simulink model "DGM_test_sim"  (R2020a)
settings: Solver=VariableStepAuto  StartTime=0.0  StopTime=smax  MaxStep=0.01  RelTol=1e-3
values from neighbouring files (symbols this model uses):
  a1 = 2    [OvereniDGMIGM.m]    (also in setup.m)
  a2 = 1.5    [OvereniDGMIGM.m]    (also in setup.m)
  a3 = 0.5    [OvereniDGMIGM.m]    (also in setup.m)
  T_1_0 = [cos(theta10), -sin(theta10), 0, a1*cos(theta10) ... (first row only)    [OvereniDGMIGM.m]    (also in setup.m)
  T_2_1 = [cos(theta20), -sin(theta20), 0, a2*cos(theta20) ... (first row only)    [OvereniDGMIGM.m]    (also in setup.m)
  T_3_2 = [cos(theta30), -sin(theta30), 0, a3*cos(theta30) ... (first row only)    [OvereniDGMIGM.m]    (also in setup.m)
undefined symbols (not defined in the file or in its folder): fi_s, fi_sample, r, R, smax, X, Y, Z
libraries: sm_lib x114, nesl_utility x58, simulink x4
(part 4 of 4)

== matlab function DGM_test_sim/MATLAB Function7 ==
  data: theta1 input; theta2 input; theta3 input; theta1_dot input; theta2_dot input; theta3_dot input; theta1_dot_dot input; theta2_dot_dot input; theta3_dot_dot input; a1 parameter; a2 parameter; a3 parameter; x output; y output; phi output; dx output; dy output; dphi output; ddx output; ddy output; ddphi output
function [ x, y, phi, dx, dy, dphi, ddx, ddy, ddphi] = POKU(theta1,theta2, theta3, theta1_dot,theta2_dot,theta3_dot,theta1_dot_dot,theta2_dot_dot,theta3_dot_dot,a1,a2,a3)
    % poloha
%     
    position = NaN(3,1);
    position(1) = a3*cos(theta1+theta2+theta3) + a2*cos(theta1+theta2) + a1*cos(theta1);
    position(2) = a3*sin(theta1+theta2+theta3) + a2*sin(theta1+theta2) + a1*sin(theta1);
    position(3) = atan2(sin(theta1+theta2+theta3),cos(theta1+theta2+theta3));
   
    % rychlost
    JQ = [-a3 * sin(theta1 + theta2 + theta3) - a2 * sin(theta1 + theta2) - a1 * sin(theta1), -a3 * sin(theta1 + theta2 + theta3) - a2 * sin(theta1 + theta2), -a3 * sin(theta1 + theta2 + theta3);
           a3 * cos(theta1 + theta2 + theta3) + a2 * cos(theta1 + theta2) + a1 * cos(theta1), a3 * cos(theta1 + theta2 + theta3) + a2 * cos(theta1 + theta2), a3 * cos(theta1 + theta2 + theta3);
          1,1,1];
    theta_dot = [theta1_dot, theta2_dot, theta3_dot]';
    theta_dot_123 = theta1_dot + theta2_dot + theta3_dot;
    theta_dot_12 = theta1_dot + theta2_dot;
    speed = JQ * theta_dot;
    
    % zrychlenis
    dJQ = [-a3 * cos(theta1 + theta1 + theta1) * theta_dot_123 - a2 * cos(theta1 + theta2) * theta_dot_12 - a1 * cos(theta1)*theta1_dot, - a3*cos(theta1 + theta2 + theta3) * theta_dot_123 - a2*cos(theta1 + theta2) * theta_dot_12, -a3 * cos(theta1 + theta2 + theta3) * theta_dot_123;
       -a3 * sin(theta1 + theta2 + theta3) * theta_dot_123 - a2 * sin(theta1 + theta2) * theta_dot_12 - a1 * sin(theta1)*theta1_dot, - a3*sin(theta1 + theta2 + theta3) * theta_dot_123 - a2*sin(theta1 + theta2) * theta_dot_12, -a3 * sin(theta1 + theta2 + theta3) * theta_dot_123;
       0,0,0];
    theta_dot_dot = [theta1_dot_dot, theta2_dot_dot, theta3_dot_dot]';

    acceleration = dJQ * theta_dot + JQ * theta_dot_dot;
    
    x = position(1);
    y = position(2);
    phi = position(3);
    dx = speed(1);
    dy = speed(2);
    dphi = speed(3);
    ddx = acceleration(1);
    ddy = acceleration(2);
    ddphi = acceleration(3);
    
end

== matlab function DGM_test_sim/MATLAB Function8 ==
  data: x input; y input; phi input; dx input; dy input; dphi input; ddx input; ddy input; ddphi input; a1 parameter; a2 parameter; a3 parameter; theta1 output size=1; theta2 output size=1; theta3 output size=1; theta1_dot output size=1; theta2_dot output size=1; theta3_dot output size=1; theta1_dot_dot output size=1; theta2_dot_dot output size=1; theta3_dot_dot output size=1
function [theta1, theta2, theta3,theta1_dot,theta2_dot,theta3_dot,theta1_dot_dot,theta2_dot_dot,theta3_dot_dot] = IOKU( x, y, phi, dx, dy, dphi, ddx, ddy, ddphi, a1, a2, a3)

% theta2
cosQ2 = ((x - a3*cos(phi))^2 + (y - a3*sin(phi))^2 - a1^2 - a2^2)/(2 * a1 * a2);
sinQ2 = -abs(sqrt(abs(1 - cosQ2^2)));
theta2 = atan2(sinQ2, cosQ2);

% theta1
A = [-a2 * sinQ2, a2 * cosQ2 + a1; a2 * cosQ2 + a1, a2 * sinQ2];
B = [x - a3*cos(phi); y - a3*sin(phi)];
X = A\B;
theta1 = atan2(X(1), X(2));

% theta3
theta3 = phi - theta1 - theta2;

% uhlova rychlost
JQ = [-a3 * sin(theta1 + theta2 + theta3) - a2 * sin(theta1 + theta2) - a1 * sin(theta1), -a3 * sin(theta1 + theta2 + theta3) - a2 * sin(theta1 + theta2), -a3 * sin(theta1 + theta2 + theta3);...
       a3 * cos(theta1 + theta2 + theta3) + a2 * cos(theta1 + theta2) + a1 * cos(theta1), a3 * cos(theta1 + theta2 + theta3) + a2 * cos(theta1 + theta2), a3 * cos(theta1 + theta2 + theta3);...
       1, 1, 1];
dX = [dx; dy; dphi];
dQ = JQ^(-1) * dX;
theta1_dot = dQ(1);
theta2_dot = dQ(2);
theta3_dot = dQ(3);

% uhlove zrychleni
dJQ = [-a3*cos(theta1+theta2+theta3)*(theta1_dot+theta2_dot+theta3_dot) - a2*cos(theta1+theta2)*(theta1_dot+theta2_dot) - a1*cos(theta1)*theta1_dot, -a3*cos(theta1+theta2+theta3)*(theta1_dot+theta2_dot+theta3_dot) - a2*cos(theta1+theta2)*(theta1_dot+theta2_dot), -a3*cos(theta1+theta2+theta3)*(theta1_dot+theta2_dot+theta3_dot);...
    -a3*sin(theta1+theta2+theta3)*(theta1_dot+theta2_dot+theta3_dot) - a2*sin(theta1+theta2)*(theta1_dot+theta2_dot) - a1*sin(theta1)*theta1_dot, -a3*sin(theta1+theta2+theta3)*(theta1_dot+theta2_dot+theta3_dot) - a2*sin(theta1+theta2)*(theta1_dot+theta2_dot), -a3*sin(theta1+theta2+theta3)*(theta1_dot+theta2_dot+theta3_dot);...
    0, 0, 0];
ddX = [ddx; ddy; ddphi];
ddQ = JQ^(-1) * (ddX - dJQ * dQ);
theta1_dot_dot = ddQ(1);
theta2_dot_dot = ddQ(2);
theta3_dot_dot = ddQ(3);


end

== matlab function DGM_test_sim/MATLAB Function10 ==
  data: x input; y input; phi input; dx input; dy input; dphi input; ddx input; ddy input; ddphi input; a1 parameter; a2 parameter; a3 parameter; theta1 output size=1; theta2 output size=1; theta3 output size=1; theta1_dot output size=1; theta2_dot output size=1; theta3_dot output size=1; theta1_dot_dot output size=1; theta2_dot_dot output size=1; theta3_dot_dot output size=1
function [theta1, theta2, theta3,theta1_dot,theta2_dot,theta3_dot,theta1_dot_dot,theta2_dot_dot,theta3_dot_dot] = IOKU( x, y, phi, dx, dy, dphi, ddx, ddy, ddphi, a1, a2, a3)

% theta2
cosQ2 = ((x - a3*cos(phi))^2 + (y - a3*sin(phi))^2 - a1^2 - a2^2)/(2 * a1 * a2);
sinQ2 = -abs(sqrt(abs(1 - cosQ2^2)));
theta2 = atan2(sinQ2, cosQ2);

% theta1
A = [-a2 * sinQ2, a2 * cosQ2 + a1; a2 * cosQ2 + a1, a2 * sinQ2];
B = [x - a3*cos(phi); y - a3*sin(phi)];
X = A\B;
theta1 = atan2(X(1), X(2));

% theta3
theta3 = phi - theta1 - theta2;

% uhlova rychlost
JQ = [-a3 * sin(theta1 + theta2 + theta3) - a2 * sin(theta1 + theta2) - a1 * sin(theta1), -a3 * sin(theta1 + theta2 + theta3) - a2 * sin(theta1 + theta2), -a3 * sin(theta1 + theta2 + theta3);...
       a3 * cos(theta1 + theta2 + theta3) + a2 * cos(theta1 + theta2) + a1 * cos(theta1), a3 * cos(theta1 + theta2 + theta3) + a2 * cos(theta1 + theta2), a3 * cos(theta1 + theta2 + theta3);...
       1, 1, 1];
dX = [dx; dy; dphi];
dQ = JQ^(-1) * dX;
theta1_dot = dQ(1);
theta2_dot = dQ(2);
theta3_dot = dQ(3);

% uhlove zrychleni
dJQ = [-a3*cos(theta1+theta2+theta3)*(theta1_dot+theta2_dot+theta3_dot) - a2*cos(theta1+theta2)*(theta1_dot+theta2_dot) - a1*cos(theta1)*theta1_dot, -a3*cos(theta1+theta2+theta3)*(theta1_dot+theta2_dot+theta3_dot) - a2*cos(theta1+theta2)*(theta1_dot+theta2_dot), -a3*cos(theta1+theta2+theta3)*(theta1_dot+theta2_dot+theta3_dot);...
    -a3*sin(theta1+theta2+theta3)*(theta1_dot+theta2_dot+theta3_dot) - a2*sin(theta1+theta2)*(theta1_dot+theta2_dot) - a1*sin(theta1)*theta1_dot, -a3*sin(theta1+theta2+theta3)*(theta1_dot+theta2_dot+theta3_dot) - a2*sin(theta1+theta2)*(theta1_dot+theta2_dot), -a3*sin(theta1+theta2+theta3)*(theta1_dot+theta2_dot+theta3_dot);...
    0, 0, 0];
ddX = [ddx; ddy; ddphi];
ddQ = JQ^(-1) * (ddX - dJQ * dQ);
theta1_dot_dot = ddQ(1);
theta2_dot_dot = ddQ(2);
theta3_dot_dot = ddQ(3);


end

== matlab function DGM_test_sim/MATLAB Function9 ==
  data: theta1 input; theta2 input; theta3 input; theta1_dot input; theta2_dot input; theta3_dot input; theta1_dot_dot input; theta2_dot_dot input; theta3_dot_dot input; a1 parameter; a2 parameter; a3 parameter; x output; y output; phi output; dx output; dy output; dphi output; ddx output; ddy output; ddphi output
function [ x, y, phi, dx, dy, dphi, ddx, ddy, ddphi] = POKU(theta1,theta2, theta3, theta1_dot,theta2_dot,theta3_dot,theta1_dot_dot,theta2_dot_dot,theta3_dot_dot,a1,a2,a3)
    % poloha
%     
    position = NaN(3,1);
    position(1) = a3*cos(theta1+theta2+theta3) + a2*cos(theta1+theta2) + a1*cos(theta1);
    position(2) = a3*sin(theta1+theta2+theta3) + a2*sin(theta1+theta2) + a1*sin(theta1);
    position(3) = atan2(sin(theta1+theta2+theta3),cos(theta1+theta2+theta3));
   
    % rychlost
    JQ = [-a3 * sin(theta1 + theta2 + theta3) - a2 * sin(theta1 + theta2) - a1 * sin(theta1), -a3 * sin(theta1 + theta2 + theta3) - a2 * sin(theta1 + theta2), -a3 * sin(theta1 + theta2 + theta3);
           a3 * cos(theta1 + theta2 + theta3) + a2 * cos(theta1 + theta2) + a1 * cos(theta1), a3 * cos(theta1 + theta2 + theta3) + a2 * cos(theta1 + theta2), a3 * cos(theta1 + theta2 + theta3);
          1,1,1];
    theta_dot = [theta1_dot, theta2_dot, theta3_dot]';
    theta_dot_123 = theta1_dot + theta2_dot + theta3_dot;
    theta_dot_12 = theta1_dot + theta2_dot;
    speed = JQ * theta_dot;
    
    % zrychlenis
    dJQ = [-a3 * cos(theta1 + theta2 + theta3) * theta_dot_123 - a2 * cos(theta1 + theta2) * theta_dot_12 - a1 * cos(theta1)*theta1_dot, - a3*cos(theta1 + theta2 + theta3) * theta_dot_123 - a2*cos(theta1 + theta2) * theta_dot_12, -a3 * cos(theta1 + theta2 + theta3) * theta_dot_123;
       -a3 * sin(theta1 + theta2 + theta3) * theta_dot_123 - a2 * sin(theta1 + theta2) * theta_dot_12 - a1 * sin(theta1)*theta1_dot, - a3*sin(theta1 + theta2 + theta3) * theta_dot_123 - a2*sin(theta1 + theta2) * theta_dot_12, -a3 * sin(theta1 + theta2 + theta3) * theta_dot_123;
       0,0,0];
    theta_dot_dot = [theta1_dot_dot, theta2_dot_dot, theta3_dot_dot]';

    acceleration = dJQ * theta_dot + JQ * theta_dot_dot;
    
    x = position(1);
    y = position(2);
    phi = position(3);
    dx = speed(1);
    dy = speed(2);
    dphi = speed(3);
    ddx = acceleration(1);
    ddy = acceleration(2);
    ddphi = acceleration(3);
    
end

== matlab function DGM_test_sim/MATLAB Function11 ==
  data: x input; y input; phi input; dx input; dy input; dphi input; ddx input; ddy input; ddphi input; a1 parameter; a2 parameter; a3 parameter; theta1 output size=1; theta2 output size=1; theta3 output size=1; theta1_dot output size=1; theta2_dot output size=1; theta3_dot output size=1; theta1_dot_dot output size=1; theta2_dot_dot output size=1; theta3_dot_dot output size=1
function [theta1, theta2, theta3,theta1_dot,theta2_dot,theta3_dot,theta1_dot_dot,theta2_dot_dot,theta3_dot_dot] = IOKU( x, y, phi, dx, dy, dphi, ddx, ddy, ddphi, a1, a2, a3)

% theta2
cosQ2 = ((x - a3*cos(phi))^2 + (y - a3*sin(phi))^2 - a1^2 - a2^2)/(2 * a1 * a2);
sinQ2 = -abs(sqrt(abs(1 - cosQ2^2)));
theta2 = atan2(sinQ2, cosQ2);

% theta1
A = [-a2 * sin(theta2), a2 * cos(theta2) + a1; a2 * cos(theta2) + a1, a2 * sin(theta2)];
B = [x - a3*cos(phi); y - a3*sin(phi)];
X = A\B;
theta1 = atan2(X(1), X(2));

% theta3
theta3 = phi - theta1 - theta2;

% uhlova rychlost
JQ = [-a3 * sin(theta1 + theta2 + theta3) - a2 * sin(theta1 + theta2) - a1 * sin(theta1), -a3 * sin(theta1 + theta2 + theta3) - a2 * sin(theta1 + theta2), -a3 * sin(theta1 + theta2 + theta3);...
       a3 * cos(theta1 + theta2 + theta3) + a2 * cos(theta1 + theta2) + a1 * cos(theta1), a3 * cos(theta1 + theta2 + theta3) + a2 * cos(theta1 + theta2), a3 * cos(theta1 + theta2 + theta3);...
       1, 1, 1];
dX = [dx; dy; dphi];
dQ = JQ^(-1) * dX;
theta1_dot = dQ(1);
theta2_dot = dQ(2);
theta3_dot = dQ(3);

% uhlove zrychleni
dJQ = [-a3*cos(theta1+theta2+theta3)*(theta1_dot+theta2_dot+theta3_dot) - a2*cos(theta1+theta2)*(theta1_dot+theta2_dot) - a1*cos(theta1)*theta1_dot, -a3*cos(theta1+theta2+theta3)*(theta1_dot+theta2_dot+theta3_dot) - a2*cos(theta1+theta2)*(theta1_dot+theta2_dot), -a3*cos(theta1+theta2+theta3)*(theta1_dot+theta2_dot+theta3_dot);...
    -a3*sin(theta1+theta2+theta3)*(theta1_dot+theta2_dot+theta3_dot) - a2*sin(theta1+theta2)*(theta1_dot+theta2_dot) - a1*sin(theta1)*theta1_dot, -a3*sin(theta1+theta2+theta3)*(theta1_dot+theta2_dot+theta3_dot) - a2*sin(theta1+theta2)*(theta1_dot+theta2_dot), -a3*sin(theta1+theta2+theta3)*(theta1_dot+theta2_dot+theta3_dot);...
    0, 0, 0];
ddX = [ddx; ddy; ddphi];
ddQ = JQ^(-1) * (ddX - dJQ * dQ);
theta1_dot_dot = ddQ(1);
theta2_dot_dot = ddQ(2);
theta3_dot_dot = ddQ(3);


end

== matlab function DGM_test_sim/MATLAB Function12 ==
  data: x input; y input; phi input; dx input; dy input; dphi input; ddx input; ddy input; ddphi input; a1 parameter; a2 parameter; a3 parameter; theta1 output size=1; theta2 output size=1; theta3 output size=1; theta1_dot output size=1; theta2_dot output size=1; theta3_dot output size=1; theta1_dot_dot output size=1; theta2_dot_dot output size=1; theta3_dot_dot output size=1
function [theta1, theta2, theta3,theta1_dot,theta2_dot,theta3_dot,theta1_dot_dot,theta2_dot_dot,theta3_dot_dot] = IOKU( x, y, phi, dx, dy, dphi, ddx, ddy, ddphi, a1, a2, a3)

% theta2
cosQ2 = ((x - a3*cos(phi))^2 + (y - a3*sin(phi))^2 - a1^2 - a2^2)/(2 * a1 * a2);
sinQ2 = -abs(sqrt(abs(1 - cosQ2^2)));
theta2 = atan2(sinQ2, cosQ2);

% theta1
A = [-a2 * sin(theta2), a2 * cos(theta2) + a1; a2 * cos(theta2) + a1, a2 * sin(theta2)];
B = [x - a3*cos(phi); y - a3*sin(phi)];
X = A\B;
theta1 = atan2(X(1), X(2));

% theta3
theta3 = phi - theta1 - theta2;

% uhlova rychlost
JQ = [-a3 * sin(theta1 + theta2 + theta3) - a2 * sin(theta1 + theta2) - a1 * sin(theta1), -a3 * sin(theta1 + theta2 + theta3) - a2 * sin(theta1 + theta2), -a3 * sin(theta1 + theta2 + theta3);...
       a3 * cos(theta1 + theta2 + theta3) + a2 * cos(theta1 + theta2) + a1 * cos(theta1), a3 * cos(theta1 + theta2 + theta3) + a2 * cos(theta1 + theta2), a3 * cos(theta1 + theta2 + theta3);...
       1, 1, 1];
dX = [dx; dy; dphi];
dQ = JQ^(-1) * dX;
theta1_dot = dQ(1);
theta2_dot = dQ(2);
theta3_dot = dQ(3);

% uhlove zrychleni
dJQ = [-a3*cos(theta1+theta2+theta3)*(theta1_dot+theta2_dot+theta3_dot) - a2*cos(theta1+theta2)*(theta1_dot+theta2_dot) - a1*cos(theta1)*theta1_dot, -a3*cos(theta1+theta2+theta3)*(theta1_dot+theta2_dot+theta3_dot) - a2*cos(theta1+theta2)*(theta1_dot+theta2_dot), -a3*cos(theta1+theta2+theta3)*(theta1_dot+theta2_dot+theta3_dot);...
    -a3*sin(theta1+theta2+theta3)*(theta1_dot+theta2_dot+theta3_dot) - a2*sin(theta1+theta2)*(theta1_dot+theta2_dot) - a1*sin(theta1)*theta1_dot, -a3*sin(theta1+theta2+theta3)*(theta1_dot+theta2_dot+theta3_dot) - a2*sin(theta1+theta2)*(theta1_dot+theta2_dot), -a3*sin(theta1+theta2+theta3)*(theta1_dot+theta2_dot+theta3_dot);...
    0, 0, 0];
ddX = [ddx; ddy; ddphi];
ddQ = JQ^(-1) * (ddX - dJQ * dQ);
theta1_dot_dot = ddQ(1);
theta2_dot_dot = ddQ(2);
theta3_dot_dot = ddQ(3);


end

== matlab function DGM_test_sim/MATLAB Function ==
  data: s input; Xstar output size=2; v input; a input; dXstar output size=2; ddXstar output size=2
function [Xstar, dXstar, ddXstar] = MCSstar(s, v, a)

    A = [2 0.5]';
    B = [-1 1]'
%     B = [1 1]';
    C = [2 2.5]'
%     sC = -A;

    r = 0.3;
    vmax = 1;
    
    if v > vmax
        v = vmax;
    else
        v = v;
    end
    nba = (A - B)/norm(A-B);
    nbc = (C-B)/norm(C-B);
    nbs = (nba+nbc)/norm(nba+nbc);
    K1 = (nba*nba'*nbs-nbs);
    l = r/(sqrt(K1'*K1));
    S = B+nbs*l;
    k = nba'*(A-S);
    Pa = A-nba*k;
    Pc = B + norm(Pa-B)*nbc;
    
%     
%     x_pab = A-k1.*nba
    Pb = B;

    helper = (Pa-S);
    fi_pa = atan2(helper(2),helper(1));
    dir = -1;
    deltafi = acos(((Pc-S)'*(Pa-S))/r^2);
    
    s1 = norm(Pa-A);
    s2 = norm(Pc-C);
    sk = r*deltafi;
    s1+s2+sk
    if s < s1
        k1 = s;
        dk1 = v;
        ddk1 = a;
        Xstar = A-k1*nba;
        dXstar = -dk1*nba;
        ddXstar = -ddk1*nba;
    elseif s1 <= s &&  s < s1+sk
        Phi = (s-s1)/r;
        dPhi = v/r;
        ddPhi = a/r;
        
        Xstar = r* [cos(fi_pa + dir*Phi); sin(fi_pa + dir*Phi)] + S;
        dXstar = r* [-sin(fi_pa + dir*Phi); cos(fi_pa + dir*Phi)]*dir*dPhi;
        ddXstar = r* [-cos(fi_pa + dir*Phi); -sin(fi_pa + dir*Phi)]*dPhi^2 + r* [-sin(fi_pa + dir*Phi); cos(fi_pa + dir*Phi)]*dir*ddPhi;
    elseif s1+sk < s && s < s1+sk+s2
        k2 = s-s1-sk;
        dk2 = v;
        ddk2 = a;
        
        Xstar = Pc + k2*nbc;
        dXstar = dk2*nbc;
        ddXstar = ddk2*nbc;
    else
%         display('ERROR V TRAJEKTORII')
        Xstar = C;
        dXstar = zeros(2,1);
        ddXstar = zeros(2,1);
    end
   
%     
%     k1 = linspace(0,norm(A-Pa),100)
% 
% 
%     
%     fi = linspace(0,deltafi,100)
%     x_rot = [r*cos(fi_pa+dir*fi);
%              r*sin(fi_pa+dir*fi)]+S
% 
%     k2 = linspace(0,norm(Pc-C),100)
%     x_pbc = Pc + k2.*nbc
% 
% 
% 
%     smax = s1+s2+sk
%     Tmax = smax/vmax
% 
%     T = 100
%     t = linspace(0,Tmax,T)
%     t1 = linspace(0,s1/vmax,T)
%     tk = linspace(s1/vmax,sk/vmax,T)
%     t2 = linspace(sk/vmax,s2/vmax,T)
%     % s = linspace(0,smax,smax/Tmax*10)
%     s = vmax*t
% 
% 
%     k1 = 0+vmax*t
% 
%     k1 = linspace(0,s1,s1/Tmax*T)
%     fi = linspace(0,(sk)/r,(sk)/Tmax*T)
%     k2 = linspace(0,s2,s2/Tmax*T)
% 
%     
%     Xk = [r*cos(fi_pa+dir*fi);r*sin(fi_pa+dir*fi)]+S
%     X2 = Pc+k2.*nbc


end

== matlab function DGM_test_sim/MATLAB Function14 ==
  data: x input; y input; phi input; dx input; dy input; dphi input; ddx input; ddy input; ddphi input; a1 parameter; a2 parameter; a3 parameter; theta1 output size=1; theta2 output size=1; theta3 output size=1; theta1_dot output size=1; theta2_dot output size=1; theta3_dot output size=1; theta1_dot_dot output size=1; theta2_dot_dot output size=1; theta3_dot_dot output size=1
function [theta1, theta2, theta3,theta1_dot,theta2_dot,theta3_dot,theta1_dot_dot,theta2_dot_dot,theta3_dot_dot] = IOKU( x, y, phi, dx, dy, dphi, ddx, ddy, ddphi, a1, a2, a3)

% theta2
cosQ2 = ((x - a3*cos(phi))^2 + (y - a3*sin(phi))^2 - a1^2 - a2^2)/(2 * a1 * a2);
sinQ2 = -abs(sqrt(abs(1 - cosQ2^2)));
theta2 = atan2(sinQ2, cosQ2);

% theta1
A = [-a2 * sin(theta2), a2 * cos(theta2) + a1; a2 * cos(theta2) + a1, a2 * sin(theta2)];
B = [x - a3*cos(phi); y - a3*sin(phi)];
X = A\B;
theta1 = atan2(X(1), X(2));

% theta3
theta3 = phi - theta1 - theta2;

% uhlova rychlost
JQ = [-a3 * sin(theta1 + theta2 + theta3) - a2 * sin(theta1 + theta2) - a1 * sin(theta1), -a3 * sin(theta1 + theta2 + theta3) - a2 * sin(theta1 + theta2), -a3 * sin(theta1 + theta2 + theta3);...
       a3 * cos(theta1 + theta2 + theta3) + a2 * cos(theta1 + theta2) + a1 * cos(theta1), a3 * cos(theta1 + theta2 + theta3) + a2 * cos(theta1 + theta2), a3 * cos(theta1 + theta2 + theta3);...
       1, 1, 1];
dX = [dx; dy; dphi];
dQ = JQ^(-1) * dX;
theta1_dot = dQ(1);
theta2_dot = dQ(2);
theta3_dot = dQ(3);

% uhlove zrychleni
dJQ = [-a3*cos(theta1+theta2+theta3)*(theta1_dot+theta2_dot+theta3_dot) - a2*cos(theta1+theta2)*(theta1_dot+theta2_dot) - a1*cos(theta1)*theta1_dot, -a3*cos(theta1+theta2+theta3)*(theta1_dot+theta2_dot+theta3_dot) - a2*cos(theta1+theta2)*(theta1_dot+theta2_dot), -a3*cos(theta1+theta2+theta3)*(theta1_dot+theta2_dot+theta3_dot);...
    -a3*sin(theta1+theta2+theta3)*(theta1_dot+theta2_dot+theta3_dot) - a2*sin(theta1+theta2)*(theta1_dot+theta2_dot) - a1*sin(theta1)*theta1_dot, -a3*sin(theta1+theta2+theta3)*(theta1_dot+theta2_dot+theta3_dot) - a2*sin(theta1+theta2)*(theta1_dot+theta2_dot), -a3*sin(theta1+theta2+theta3)*(theta1_dot+theta2_dot+theta3_dot);...
    0, 0, 0];
ddX = [ddx; ddy; ddphi];
ddQ = JQ^(-1) * (ddX - dJQ * dQ);
theta1_dot_dot = ddQ(1);
theta2_dot_dot = ddQ(2);
theta3_dot_dot = ddQ(3);


end

== matlab function DGM_test_sim/MATLAB Function15 ==
  data: s input; Xstar output size=2; v input; a input; dXstar output size=2; ddXstar output size=2
function [Xstar, dXstar, ddXstar] = MCSstar(s, v, a)

    A = [2 0.5]';
    B = [0 1]';
%     B = [1 1]';
    C = [2 2.5]';
%     sC = -A;

    r = 0.3;
    vmax = 1;
    
    if v > vmax
        v = vmax;
    else
        v = v;
    end
    nba = (A - B)/norm(A-B);
    nbc = (C-B)/norm(C-B);
    nbs = (nba+nbc)/norm(nba+nbc);
    K1 = (nba*nba'*nbs-nbs);
    l = r/(sqrt(K1'*K1));
    S = B+nbs*l;
    k = nba'*(A-S);
    Pa = A-nba*k;
    Pc = B + norm(Pa-B)*nbc;
    
%     
%     x_pab = A-k1.*nba
    Pb = B;

    helper = (Pa-S);
    fi_pa = atan2(helper(2),helper(1));
    dir = -1;
    deltafi = acos(((Pc-S)'*(Pa-S))/r^2);
    
    s1 = norm(Pa-A);
    s2 = norm(Pc-C);
    sk = r*deltafi;
    s1+s2+sk;
    if s < s1
        k1 = s;
        dk1 = v;
        ddk1 = a;
        Xstar = A-k1*nba;
        dXstar = -dk1*nba;
        ddXstar = -ddk1*nba;
    elseif s1 <= s &&  s < s1+sk
        Phi = (s-s1)/r;
        dPhi = v/r;
        ddPhi = a/r;
        
        Xstar = r* [cos(fi_pa + dir*Phi); sin(fi_pa + dir*Phi)] + S;
        dXstar = r* [-sin(fi_pa + dir*Phi); cos(fi_pa + dir*Phi)]*dir*dPhi;
        ddXstar = r* [-cos(fi_pa + dir*Phi); -sin(fi_pa + dir*Phi)]*dPhi^2 + r* [-sin(fi_pa + dir*Phi); cos(fi_pa + dir*Phi)]*dir*ddPhi;
    elseif s1+sk < s && s < s1+sk+s2
        k2 = s-s1-sk;
        dk2 = v;
        ddk2 = a;
        
        Xstar = Pc + k2*nbc;
        dXstar = dk2*nbc;
        ddXstar = ddk2*nbc;
    else
%         display('ERROR V TRAJEKTORII')
        Xstar = C;
        dXstar = zeros(2,1);
        ddXstar = zeros(2,1);
    end
   
%     
%     k1 = linspace(0,norm(A-Pa),100)
% 
% 
%     
%     fi = linspace(0,deltafi,100)
%     x_rot = [r*cos(fi_pa+dir*fi);
%              r*sin(fi_pa+dir*fi)]+S
% 
%     k2 = linspace(0,norm(Pc-C),100)
%     x_pbc = Pc + k2.*nbc
% 
% 
% 
%     smax = s1+s2+sk
%     Tmax = smax/vmax
% 
%     T = 100
%     t = linspace(0,Tmax,T)
%     t1 = linspace(0,s1/vmax,T)
%     tk = linspace(s1/vmax,sk/vmax,T)
%     t2 = linspace(sk/vmax,s2/vmax,T)
%     % s = linspace(0,smax,smax/Tmax*10)
%     s = vmax*t
% 
% 
%     k1 = 0+vmax*t
% 
%     k1 = linspace(0,s1,s1/Tmax*T)
%     fi = linspace(0,(sk)/r,(sk)/Tmax*T)
%     k2 = linspace(0,s2,s2/Tmax*T)
% 
%     
%     Xk = [r*cos(fi_pa+dir*fi);r*sin(fi_pa+dir*fi)]+S
%     X2 = Pc+k2.*nbc


end

== matlab function DGM_test_sim/MATLAB Function1 ==
  data: theta1 output size=1; x input; theta2 output size=1; y input; phi input; a1 input; a2 input; a3 input; theta3 output size=1
function [theta1, theta2, theta3] = IGM( x, y, phi, a1, a2, a3)
    cosQ2 = ((x - a3 *cos(phi))^2 + (y - a3 * sin(phi))^2 - a2^2 - a1^2)/(2*a1*a2);
    sinQ2 =  -abs(sqrt(abs(1 - cosQ2^2))); % 2 reseni, vybereme -
    
    theta2 = atan2(sinQ2, cosQ2); % Q2
%     A = [-a2 * sin(theta2), a2*cos(theta2) + a1;
%          a2 * cos(theta2)  + a1, a2*sin(theta2)];
     A = [-a2 * sinQ2, a2*cosQ2 + a1;
         a2 * cosQ2  + a1, a2*sinQ2];
    b = [x - a3 * cos(phi); y - a3 * sin(phi)];
    
    X = inv(A)*b;
%     sin(theta1) = X(1);
%     cos(theta1) = X(2);
    
    theta1 = atan2(X(1),X(2)); % Q1
    
    theta3 = mod(phi - theta2 - theta1,2*pi); % Q3
end

== matlab function DGM_test_sim/MATLAB Function6 ==
  data: Q1 output size=1; x input; Q2 output size=1; y input; phi input; Q3 output size=1; a1 parameter; a2 parameter; a3 parameter
function [Q1, Q2, Q3] = IGM( x, y, phi, a1, a2, a3)
    cosQ2 = ((x - a3 *cos(phi))^2 + (y - a3 * sin(phi))^2 - a2^2 - a1^2)/(2*a1*a2);
    sinQ2 =  -abs(sqrt(abs(1 - cosQ2^2))); % 2 reseni, vybereme -
    
    Q2 = atan2(sinQ2, cosQ2); % Q2
%     A = [-a2 * sin(theta2), a2*cos(theta2) + a1;
%          a2 * cos(theta2)  + a1, a2*sin(theta2)];
     A = [-a2 * sinQ2, a2*cosQ2 + a1;
         a2 * cosQ2  + a1, a2*sinQ2];
    b = [x - a3 * cos(phi); y - a3 * sin(phi)];
    
    X = inv(A)*b;
%     sin(theta1) = X(1);
%     cos(theta1) = X(2);
    
    Q1 = atan2(X(1),X(2)); % Q1
    
    Q3 = mod(phi - Q2 - Q1,2*pi); % Q3
end

== matlab function DGM_test_sim/MATLAB Function2 ==
  data: x output; theta1 input; y output; theta2 input; theta3 input; a1 input; a2 input; a3 input; phi output
function [x,y,phi] = DGM(theta1, theta2, theta3,a1,a2,a3)
   x = a3*cos(theta1+theta2+theta3) + a2*cos(theta1+theta2) + a1*cos(theta1);
   y = a3*sin(theta1+theta2+theta3) + a2*sin(theta1+theta2) + a1*sin(theta1);
   phi = atan2(sin(theta1+theta2+theta3),cos(theta1+theta2+theta3));
%    phi2 = theta1+theta2+theta3
end

== matlab function DGM_test_sim/MATLAB Function3 ==
  data: x output; theta1 input; y output; theta2 input; theta3 input; a1 input; a2 input; a3 input; phi output
function [x,y,phi] = DGM(theta1, theta2, theta3,a1,a2,a3)
   x = a3*cos(theta1+theta2+theta3) + a2*cos(theta1+theta2) + a1*cos(theta1);
   y = a3*sin(theta1+theta2+theta3) + a2*sin(theta1+theta2) + a1*sin(theta1);
   phi = atan2(sin(theta1+theta2+theta3),cos(theta1+theta2+theta3));
%    phi2 = theta1+theta2+theta3
end

== matlab function DGM_test_sim/MATLAB Function4 ==
  data: theta1 output size=1; x input; theta2 output size=1; y input; phi input; a1 input; a2 input; a3 input; theta3 output size=1
function [theta1, theta2, theta3] = IGM( x, y, phi, a1, a2, a3)
    cosQ2 = ((x - a3 *cos(phi))^2 + (y - a3 * sin(phi))^2 - a2^2 - a1^2)/(2*a1*a2);
    sinQ2 =  -abs(sqrt(abs(1 - cosQ2^2))); % 2 reseni, vybereme -
    
    theta2 = atan2(sinQ2, cosQ2); % Q2
%     A = [-a2 * sin(theta2), a2*cos(theta2) + a1;
%          a2 * cos(theta2)  + a1, a2*sin(theta2)];
     A = [-a2 * sinQ2, a2*cosQ2 + a1;
         a2 * cosQ2  + a1, a2*sinQ2];
    b = [x - a3 * cos(phi); y - a3 * sin(phi)];
    
    X = inv(A)*b;
%     sin(theta1) = X(1);
%     cos(theta1) = X(2);
    
    theta1 = atan2(X(1),X(2)); % Q1
    
    theta3 = mod(phi - theta2 - theta1,2*pi); % Q3
end
